simulink model "fixedphone"  (Simulink 6.3)
settings: Solver=ode45  StartTime=0.0  StopTime=10.0  RelTol=1e-3
libraries: simulink x10
settings Model: LastModifiedBy=hnine

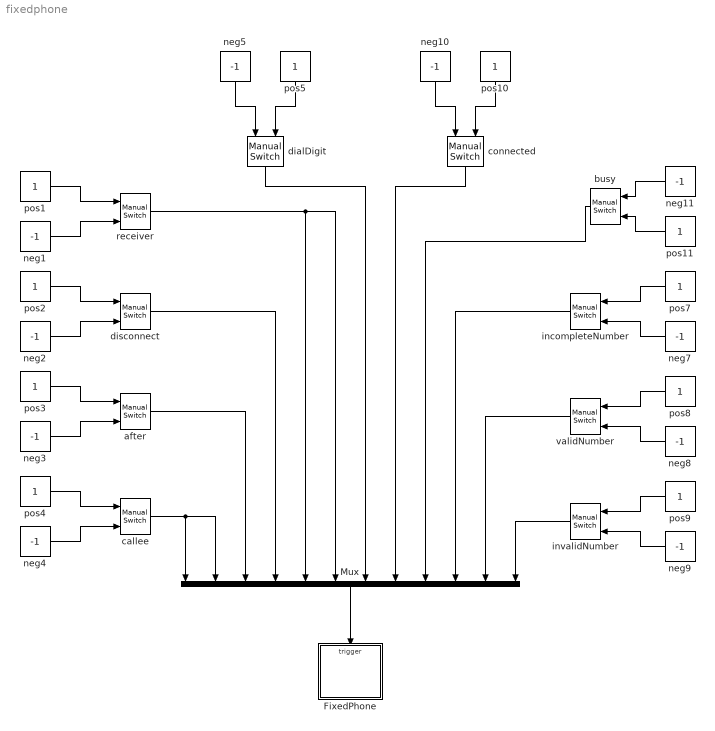
== system fixedphone ==
  FixedPhone : Stateflow chart  TreatAsAtomicUnit=on
  Mux : Mux  Orientation=down  Inputs=12
  after : simulink/Signal Routing/Manual Switch  sw=1  action=0
  busy : simulink/Signal Routing/Manual Switch  Orientation=left  sw=1  action=0
  callee : simulink/Signal Routing/Manual Switch  sw=1  action=0
  connected : simulink/Signal Routing/Manual Switch  Orientation=down  sw=1  action=0
  dialDigit : simulink/Signal Routing/Manual Switch  Orientation=down  sw=1  action=0
  disconnect : simulink/Signal Routing/Manual Switch  sw=1  action=0
  incompleteNumber : simulink/Signal Routing/Manual Switch  Orientation=left  sw=1  action=0
  invalidNumber : simulink/Signal Routing/Manual Switch  Orientation=left  sw=1  action=0
  neg{1..4} (4 alike) : Constant  Value=-1
  neg10 : Constant  Orientation=down  Value=-1
  neg{7..9,11} (4 alike) : Constant  Orientation=left  Value=-1
  neg5 : Constant  Orientation=down  Value=-1
  pos{1..4} (4 alike) : Constant
  pos10 : Constant  Orientation=down
  pos{7..9,11} (4 alike) : Constant  Orientation=left
  pos5 : Constant  Orientation=down
  receiver : simulink/Signal Routing/Manual Switch  sw=0  action=0
  validNumber : simulink/Signal Routing/Manual Switch  Orientation=left  sw=1  action=0
  wires:
  pos1/1 -> receiver/1
  neg1/1 -> receiver/2
  pos2/1 -> disconnect/1
  neg2/1 -> disconnect/2
  pos3/1 -> after/1
  neg3/1 -> after/2
  pos4/1 -> callee/1
  neg4/1 -> callee/2
  neg5/1 -> dialDigit/1
  pos5/1 -> dialDigit/2
  pos7/1 -> incompleteNumber/1
  neg7/1 -> incompleteNumber/2
  pos8/1 -> validNumber/1
  neg8/1 -> validNumber/2
  pos9/1 -> invalidNumber/1
  neg9/1 -> invalidNumber/2
  neg10/1 -> connected/1
  pos10/1 -> connected/2
  neg11/1 -> busy/1
  pos11/1 -> busy/2
  callee/1 -> Mux/1, Mux/2
  after/1 -> Mux/3
  disconnect/1 -> Mux/4
  receiver/1 -> Mux/5, Mux/6
  dialDigit/1 -> Mux/7
  connected/1 -> Mux/8
  busy/1 -> Mux/9
  incompleteNumber/1 -> Mux/10
  validNumber/1 -> Mux/11
  invalidNumber/1 -> Mux/12
  Mux/1 -> FixedPhone/Trigger

== stateflow chart FixedPhone ==
  state Idle
    en: idling()
    state idling [function]
      (default) -> (junction 34) : { System.out.println( "I'm idling around" ); }
  state Active
    en: turnOnDisplay()
    ex: turnOffDisplay()
    state DialTone
      du: playDialTone()
      state playDialTone [function]
        (default) -> (junction 33) : { System.out.println( "rrrrrrrrrrrr.." ); }
    state Timeout
      du: playMessage()
      state playMessage [function]
        (default) -> (junction 29) : { System.out.println("timeout, please hang up and try again"); }
    state Dialing
      state Send
      state Wait
      state Receive
      Wait -> Send : dialDigit
      Send -> Receive
      Receive -> Wait [order 3] : incompleteNumber
    state Invalid
      du: playMessage()
      state playMessage [function]
        (default) -> (junction 30) : { System.out.println( "invalid number" ); }
    state Connecting
      en: System.out.println( "connecting.." );
    state Busy
      du: playBusyTone()
      state playBusyTone [function]
        (default) -> (junction 31) : { System.out.println( "beep beep beep.." ); }
    state Ringing
      du: playRingTone()
      state enableSpeech [function]
        (default) -> (junction 28) : { System.out.println( "enable speech" ); }
      state playRingTone [function]
        (default) -> (junction 32) : { System.out.println( "rring, rring .." ); }
    state Talking
    state Pinned
    state turnOnDisplay [function]
      (default) -> (junction 26) : { System.out.println( "display on" ); }
    state turnOffDisplay [function]
      (default) -> (junction 27) : { System.out.println( "display off" ); }
    (default) -> DialTone
    DialTone -> Timeout [order 1] : after
    DialTone -> Send [order 2] : dialDigit
    Dialing -> Timeout : after
    Receive -> Invalid [order 1] : invalidNumber
    Receive -> Connecting [order 2] : validNumber
    Connecting -> Busy [order 1] : busy
    Ringing -> Talking : calleeAnswers
        | /enableSpeech()
    Talking -> Pinned : calleeHangsUp
    Pinned -> Talking : calleeAnswers
    Connecting -> Ringing [order 2] : connected
  (default) -> Idle
  Idle -> Active : liftReceiver
      | /System.out.println( "lifted receiver" );
  Active -> Idle [order 1] : hangupReceiver
  Active -> Active [order 2] : disconnect
  events: calleeAnswers input RISING_EDGE_EVENT; calleeHangsUp input FALLING_EDGE_EVENT; after input EITHER_EDGE_EVENT; disconnect input EITHER_EDGE_EVENT; liftReceiver input RISING_EDGE_EVENT; hangupReceiver input FALLING_EDGE_EVENT; dialDigit input EITHER_EDGE_EVENT; connected input EITHER_EDGE_EVENT; busy input EITHER_EDGE_EVENT; checkNumber input EITHER_EDGE_EVENT; incompleteNumber input EITHER_EDGE_EVENT; validNumber input EITHER_EDGE_EVENT; invalidNumber input EITHER_EDGE_EVENT
